simulink model "gm_uz_pmsm_model"  (R2023b)
settings: Solver=FixedStepAuto  StartTime=0.0  StopTime=0.05  RelTol=1e-3
PreLoadFcn:
  | uz_pmsm_model_init_parameter
PostLoadFcn:
  | % Import the data from Excel for a lookup table
  | FluxMapData = readtable('C:\Users\Philipp\ultrazohm\ultrazohm_sw\ip_cores\uz_pmsm_model\FluxMapData_2023-05-26_13-07-57.csv');
  | % Row indices for lookup table
  | d_current_in_d_axis = FluxMapData(8:27,1:end);
  | % Column indices for lookup table
  | q_current_in_d_axis = FluxMapData(29:48,1:end);
  | % Output values for lookup table
  | d_Flux_d_axis = FluxMapData(50:69,1:end);
undefined symbols (not defined in the file or in its folder): ad1, ad2, ad3, ad4, ad5, ad6, aq1, aq2, aq3, aq4, aq5, aq6, d_current_d_Flux, d_current_q_Flux, entkopplung_dynamic, entkopplung_linear, entkopplung_static, Fid1_Giq1, Fid2_Giq2, Flux_d, Flux_q, friction_coefficient, inertia, Ki_Bo_d, Ki_Bo_q, Kp_Bo_d, Kp_Bo_q, L_d, L_q, Ldq, parameter_nachfuerung, polepair, praediktion_entkopplung_nonlinear, psi_pm, q_current_d_Flux, q_current_q_Flux, R_1, simulate_mechanical, simulate_nonlinear_modell, simulate_open_loop, static_friction_torque, tau_sum, ts_regler
libraries: hdlmdlgenlib x21, slpidlib x6
(part 4 of 4)

== system gm_uz_pmsm_model/uz_pmsm_model/Sum23 ==
  In1 : Inport
  In2 : Inport  Port=2
  Sum23 : Sum  Inputs=+-  OutDataTypeStr=single  SampleTime=1e-08
  Sum23_pd1 : Delay  DelayLength=6
  Out1 : Outport
  wires:
  In1/1 -> Sum23/1
  In2/1 -> Sum23/2
  Sum23/1 -> Sum23_pd1/1
  Sum23_pd1/1 -> Out1/1

== system gm_uz_pmsm_model/uz_pmsm_model/Sum3 ==
  In1 : Inport
  In2 : Inport  Port=2
  Sum3 : Sum  Inputs=+-  OutDataTypeStr=single  SampleTime=1e-08
  Sum3_pd1 : Delay  DelayLength=6
  Out1 : Outport
  wires:
  In1/1 -> Sum3/1
  In2/1 -> Sum3/2
  Sum3/1 -> Sum3_pd1/1
  Sum3_pd1/1 -> Out1/1

== system gm_uz_pmsm_model/uz_pmsm_model/Sum31 ==
  In1 : Inport
  In2 : Inport  Port=2
  Sum31 : Sum  Inputs=+-  OutDataTypeStr=single  SampleTime=1e-08
  Sum31_pd1 : Delay  DelayLength=6
  Out1 : Outport
  wires:
  In1/1 -> Sum31/1
  In2/1 -> Sum31/2
  Sum31/1 -> Sum31_pd1/1
  Sum31_pd1/1 -> Out1/1

== system gm_uz_pmsm_model/uz_pmsm_model/Sum32 ==
  In1 : Inport
  In2 : Inport  Port=2
  Sum32 : Sum  OutDataTypeStr=single  SampleTime=1e-08
  Sum32_pd1 : Delay  DelayLength=6
  Out1 : Outport
  wires:
  In1/1 -> Sum32/1
  In2/1 -> Sum32/2
  Sum32/1 -> Sum32_pd1/1
  Sum32_pd1/1 -> Out1/1

== system gm_uz_pmsm_model/uz_pmsm_model/Sum33 ==
  In1 : Inport
  In2 : Inport  Port=2
  Sum33 : Sum  Inputs=+-  OutDataTypeStr=single  SampleTime=1e-08
  Sum33_pd1 : Delay  DelayLength=6
  Out1 : Outport
  wires:
  In1/1 -> Sum33/1
  In2/1 -> Sum33/2
  Sum33/1 -> Sum33_pd1/1
  Sum33_pd1/1 -> Out1/1

== system gm_uz_pmsm_model/uz_pmsm_model/Sum3_stage2 ==
  In1 : Inport
  In2 : Inport  Port=2
  Sum3_stage2 : Sum  OutDataTypeStr=single  SampleTime=1e-08
  Sum3_stage2_pd1 : Delay  DelayLength=6
  Out1 : Outport
  wires:
  In1/1 -> Sum3_stage2/1
  In2/1 -> Sum3_stage2/2
  Sum3_stage2/1 -> Sum3_stage2_pd1/1
  Sum3_stage2_pd1/1 -> Out1/1

== system gm_uz_pmsm_model/uz_pmsm_model/Sum3_stage21 ==
  In1 : Inport
  In2 : Inport  Port=2
  Sum3_stage21 : Sum  Inputs=+-  OutDataTypeStr=single  SampleTime=1e-08
  Sum3_stage21_pd1 : Delay  DelayLength=6
  Out1 : Outport
  wires:
  In1/1 -> Sum3_stage21/1
  In2/1 -> Sum3_stage21/2
  Sum3_stage21/1 -> Sum3_stage21_pd1/1
  Sum3_stage21_pd1/1 -> Out1/1

== system gm_uz_pmsm_model/uz_pmsm_model/Sum3_stage3 ==
  In1 : Inport
  In2 : Inport  Port=2
  Sum3_stage3 : Sum  Inputs=+-  OutDataTypeStr=single  SampleTime=1e-08
  Sum3_stage3_pd1 : Delay  DelayLength=6
  Out1 : Outport
  wires:
  In1/1 -> Sum3_stage3/1
  In2/1 -> Sum3_stage3/2
  Sum3_stage3/1 -> Sum3_stage3_pd1/1
  Sum3_stage3_pd1/1 -> Out1/1

== system gm_uz_pmsm_model/uz_pmsm_model/Sum3_stage31 ==
  In1 : Inport
  In2 : Inport  Port=2
  Sum3_stage31 : Sum  Inputs=+-  OutDataTypeStr=single  SampleTime=1e-08
  Sum3_stage31_pd1 : Delay  DelayLength=6
  Out1 : Outport
  wires:
  In1/1 -> Sum3_stage31/1
  In2/1 -> Sum3_stage31/2
  Sum3_stage31/1 -> Sum3_stage31_pd1/1
  Sum3_stage31_pd1/1 -> Out1/1

== system gm_uz_pmsm_model/uz_pmsm_model/Sum3_stage4 ==
  In1 : Inport
  In2 : Inport  Port=2
  Sum3_stage4 : Sum  OutDataTypeStr=single  SampleTime=1e-08
  Sum3_stage4_pd1 : Delay  DelayLength=6
  Out1 : Outport
  wires:
  In1/1 -> Sum3_stage4/1
  In2/1 -> Sum3_stage4/2
  Sum3_stage4/1 -> Sum3_stage4_pd1/1
  Sum3_stage4_pd1/1 -> Out1/1

== system gm_uz_pmsm_model/uz_pmsm_model/Sum4 ==
  In1 : Inport
  In2 : Inport  Port=2
  Sum4 : Sum  Inputs=+-  OutDataTypeStr=single  SampleTime=1e-08
  Sum4_pd1 : Delay  DelayLength=6
  Out1 : Outport
  wires:
  In1/1 -> Sum4/1
  In2/1 -> Sum4/2
  Sum4/1 -> Sum4_pd1/1
  Sum4_pd1/1 -> Out1/1

== system gm_uz_pmsm_model/uz_pmsm_model/Sum41 ==
  In1 : Inport
  In2 : Inport  Port=2
  Sum41 : Sum  OutDataTypeStr=single  SampleTime=1e-08
  Sum41_pd1 : Delay  DelayLength=6
  Out1 : Outport
  wires:
  In1/1 -> Sum41/1
  In2/1 -> Sum41/2
  Sum41/1 -> Sum41_pd1/1
  Sum41_pd1/1 -> Out1/1

== system gm_uz_pmsm_model/uz_pmsm_model/Sum42 ==
  In1 : Inport
  In2 : Inport  Port=2
  Sum42 : Sum  OutDataTypeStr=single  SampleTime=1e-08
  Sum42_pd1 : Delay  DelayLength=6
  Out1 : Outport
  wires:
  In1/1 -> Sum42/1
  In2/1 -> Sum42/2
  Sum42/1 -> Sum42_pd1/1
  Sum42_pd1/1 -> Out1/1

== system gm_uz_pmsm_model/uz_pmsm_model/Sum4_stage2 ==
  In1 : Inport
  In2 : Inport  Port=2
  Sum4_stage2 : Sum  Inputs=+-  OutDataTypeStr=single  SampleTime=1e-08
  Sum4_stage2_pd1 : Delay  DelayLength=6
  Out1 : Outport
  wires:
  In1/1 -> Sum4_stage2/1
  In2/1 -> Sum4_stage2/2
  Sum4_stage2/1 -> Sum4_stage2_pd1/1
  Sum4_stage2_pd1/1 -> Out1/1

== system gm_uz_pmsm_model/uz_pmsm_model/Sum4_stage3 ==
  In1 : Inport
  In2 : Inport  Port=2
  Sum4_stage3 : Sum  Inputs=+-  OutDataTypeStr=single  SampleTime=1e-08
  Sum4_stage3_pd1 : Delay  DelayLength=6
  Out1 : Outport
  wires:
  In1/1 -> Sum4_stage3/1
  In2/1 -> Sum4_stage3/2
  Sum4_stage3/1 -> Sum4_stage3_pd1/1
  Sum4_stage3_pd1/1 -> Out1/1

== system gm_uz_pmsm_model/uz_pmsm_model/Sum4_stage4 ==
  In1 : Inport
  In2 : Inport  Port=2
  Sum4_stage4 : Sum  Inputs=+-  OutDataTypeStr=single  SampleTime=1e-08
  Sum4_stage4_pd1 : Delay  DelayLength=6
  Out1 : Outport
  wires:
  In1/1 -> Sum4_stage4/1
  In2/1 -> Sum4_stage4/2
  Sum4_stage4/1 -> Sum4_stage4_pd1/1
  Sum4_stage4_pd1/1 -> Out1/1

== system gm_uz_pmsm_model/uz_pmsm_model/Sum5 ==
  In1 : Inport
  In2 : Inport  Port=2
  Sum5 : Sum  Inputs=+-  OutDataTypeStr=single  SampleTime=1e-08
  Sum5_pd1 : Delay  DelayLength=6
  Out1 : Outport
  wires:
  In1/1 -> Sum5/1
  In2/1 -> Sum5/2
  Sum5/1 -> Sum5_pd1/1
  Sum5_pd1/1 -> Out1/1

== system gm_uz_pmsm_model/uz_pmsm_model/Sum51 ==
  In1 : Inport
  In2 : Inport  Port=2
  Sum51 : Sum  OutDataTypeStr=single  SampleTime=1e-08
  Sum51_pd1 : Delay  DelayLength=6
  Out1 : Outport
  wires:
  In1/1 -> Sum51/1
  In2/1 -> Sum51/2
  Sum51/1 -> Sum51_pd1/1
  Sum51_pd1/1 -> Out1/1

== system gm_uz_pmsm_model/uz_pmsm_model/Sum52 ==
  In1 : Inport
  In2 : Inport  Port=2
  Sum52 : Sum  OutDataTypeStr=single  SampleTime=1e-08
  Sum52_pd1 : Delay  DelayLength=6
  Out1 : Outport
  wires:
  In1/1 -> Sum52/1
  In2/1 -> Sum52/2
  Sum52/1 -> Sum52_pd1/1
  Sum52_pd1/1 -> Out1/1

== system gm_uz_pmsm_model/uz_pmsm_model/Sum53 ==
  In1 : Inport
  In2 : Inport  Port=2
  Sum53 : Sum  OutDataTypeStr=single  SampleTime=1e-08
  Sum53_pd1 : Delay  DelayLength=6
  Out1 : Outport
  wires:
  In1/1 -> Sum53/1
  In2/1 -> Sum53/2
  Sum53/1 -> Sum53_pd1/1
  Sum53_pd1/1 -> Out1/1

== system gm_uz_pmsm_model/uz_pmsm_model/Sum6 ==
  In1 : Inport
  In2 : Inport  Port=2
  Sum6 : Sum  Inputs=+-  OutDataTypeStr=single  SampleTime=1e-08
  Sum6_pd1 : Delay  DelayLength=6
  Out1 : Outport
  wires:
  In1/1 -> Sum6/1
  In2/1 -> Sum6/2
  Sum6/1 -> Sum6_pd1/1
  Sum6_pd1/1 -> Out1/1

== system gm_uz_pmsm_model/uz_pmsm_model/Sum7 ==
  In1 : Inport
  In2 : Inport  Port=2
  Sum7 : Sum  Inputs=+-  OutDataTypeStr=single  SampleTime=1e-08
  Sum7_pd1 : Delay  DelayLength=6
  Out1 : Outport
  wires:
  In1/1 -> Sum7/1
  In2/1 -> Sum7/2
  Sum7/1 -> Sum7_pd1/1
  Sum7_pd1/1 -> Out1/1

== system gm_uz_pmsm_model/uz_pmsm_model/Sum71 ==
  In1 : Inport
  In2 : Inport  Port=2
  Sum71 : Sum  Inputs=+-  OutDataTypeStr=single  SampleTime=1e-08
  Sum71_pd1 : Delay  DelayLength=6
  Out1 : Outport
  wires:
  In1/1 -> Sum71/1
  In2/1 -> Sum71/2
  Sum71/1 -> Sum71_pd1/1
  Sum71_pd1/1 -> Out1/1

== system gm_uz_pmsm_model/uz_pmsm_model/Sum8 ==
  In1 : Inport
  In2 : Inport  Port=2
  Sum8 : Sum  Inputs=+-  OutDataTypeStr=single  SampleTime=1e-08
  Sum8_pd1 : Delay  DelayLength=6
  Out1 : Outport
  wires:
  In1/1 -> Sum8/1
  In2/1 -> Sum8/2
  Sum8/1 -> Sum8_pd1/1
  Sum8_pd1/1 -> Out1/1

== system gm_uz_pmsm_model/uz_pmsm_model/Tanh ==
  In1 : Inport
  Tanh : Trigonometry  Operator=tanh  SampleTime=1e-08
  Tanh_pd1 : Delay  DelayLength=25
  Out1 : Outport
  wires:
  In1/1 -> Tanh/1
  Tanh/1 -> Tanh_pd1/1
  Tanh_pd1/1 -> Out1/1

== system gm_uz_pmsm_model/uz_pmsm_model/Tanh1 ==
  In1 : Inport
  Tanh1 : Trigonometry  Operator=cosh  SampleTime=1e-08
  Tanh1_pd1 : Delay  DelayLength=17
  Out1 : Outport
  wires:
  In1/1 -> Tanh1/1
  Tanh1/1 -> Tanh1_pd1/1
  Tanh1_pd1/1 -> Out1/1

== system gm_uz_pmsm_model/uz_pmsm_model/Tanh11 ==
  In1 : Inport
  Tanh11 : Trigonometry  Operator=tanh  SampleTime=1e-08
  Tanh11_pd1 : Delay  DelayLength=25
  Out1 : Outport
  wires:
  In1/1 -> Tanh11/1
  Tanh11/1 -> Tanh11_pd1/1
  Tanh11_pd1/1 -> Out1/1

== system gm_uz_pmsm_model/uz_pmsm_model/Tanh12 ==
  In1 : Inport
  Tanh12 : Trigonometry  Operator=tanh  SampleTime=1e-08
  Tanh12_pd1 : Delay  DelayLength=25
  Out1 : Outport
  wires:
  In1/1 -> Tanh12/1
  Tanh12/1 -> Tanh12_pd1/1
  Tanh12_pd1/1 -> Out1/1

== system gm_uz_pmsm_model/uz_pmsm_model/Tanh13 ==
  In1 : Inport
  Tanh13 : Trigonometry  Operator=cosh  SampleTime=1e-08
  Tanh13_pd1 : Delay  DelayLength=17
  Out1 : Outport
  wires:
  In1/1 -> Tanh13/1
  Tanh13/1 -> Tanh13_pd1/1
  Tanh13_pd1/1 -> Out1/1

== system gm_uz_pmsm_model/uz_pmsm_model/Tanh2 ==
  In1 : Inport
  Tanh2 : Trigonometry  Operator=cosh  SampleTime=1e-08
  Tanh2_pd1 : Delay  DelayLength=17
  Out1 : Outport
  wires:
  In1/1 -> Tanh2/1
  Tanh2/1 -> Tanh2_pd1/1
  Tanh2_pd1/1 -> Out1/1

== system gm_uz_pmsm_model/uz_pmsm_model/Tanh21 ==
  In1 : Inport
  Tanh21 : Trigonometry  Operator=cosh  SampleTime=1e-08
  Tanh21_pd1 : Delay  DelayLength=17
  Out1 : Outport
  wires:
  In1/1 -> Tanh21/1
  Tanh21/1 -> Tanh21_pd1/1
  Tanh21_pd1/1 -> Out1/1

== system gm_uz_pmsm_model/uz_pmsm_model/Tanh3 ==
  In1 : Inport
  Tanh3 : Trigonometry  Operator=cosh  SampleTime=1e-08
  Tanh3_pd1 : Delay  DelayLength=17
  Out1 : Outport
  wires:
  In1/1 -> Tanh3/1
  Tanh3/1 -> Tanh3_pd1/1
  Tanh3_pd1/1 -> Out1/1

== system gm_uz_pmsm_model/uz_pmsm_model/Tanh31 ==
  In1 : Inport
  Tanh31 : Trigonometry  Operator=cosh  SampleTime=1e-08
  Tanh31_pd1 : Delay  DelayLength=17
  Out1 : Outport
  wires:
  In1/1 -> Tanh31/1
  Tanh31/1 -> Tanh31_pd1/1
  Tanh31_pd1/1 -> Out1/1

== system gm_uz_pmsm_model/uz_pmsm_model/Tanh4 ==
  In1 : Inport
  Tanh4 : Trigonometry  Operator=cosh  SampleTime=1e-08
  Tanh4_pd1 : Delay  DelayLength=17
  Out1 : Outport
  wires:
  In1/1 -> Tanh4/1
  Tanh4/1 -> Tanh4_pd1/1
  Tanh4_pd1/1 -> Out1/1

== system gm_uz_pmsm_model/uz_pmsm_model/Tanh41 ==
  In1 : Inport
  Tanh41 : Trigonometry  Operator=cosh  SampleTime=1e-08
  Tanh41_pd1 : Delay  DelayLength=17
  Out1 : Outport
  wires:
  In1/1 -> Tanh41/1
  Tanh41/1 -> Tanh41_pd1/1
  Tanh41_pd1/1 -> Out1/1

== system gm_uz_pmsm_model/uz_pmsm_model/Tanh5 ==
  In1 : Inport
  Tanh5 : Trigonometry  Operator=tanh  SampleTime=1e-08
  Tanh5_pd1 : Delay  DelayLength=25
  Out1 : Outport
  wires:
  In1/1 -> Tanh5/1
  Tanh5/1 -> Tanh5_pd1/1
  Tanh5_pd1/1 -> Out1/1

== system gm_uz_pmsm_model/Curren t_Controller_With_FluxMaps_OLD/Entkopplungen/Lineare_Entkopplung ==
  i_d : Inport
  i_q : Inport  Port=2
  omega_m : Inport  Port=3
  Constant1 : Constant  Value=psi_pm  SampleTime=-1
  Gain : Gain  Gain=L_q
  Gain1 : Gain  Gain=L_d
  Gain2 : Gain  Gain=polepair
  Product : Product
  Product1 : Product
  Sum6 : Sum  Inputs=|++
  u_d : Outport
  u_q : Outport  Port=2
  wires:
  Gain/1 -> Product/1
  Gain2/1 -> Product/2, Product1/2
  Gain1/1 -> Sum6/1
  Product1/1 -> u_q/1
  i_q/1 -> Gain/1
  Constant1/1 -> Sum6/2
  i_d/1 -> Gain1/1
  Product/1 -> u_d/1
  Sum6/1 -> Product1/1
  omega_m/1 -> Gain2/1

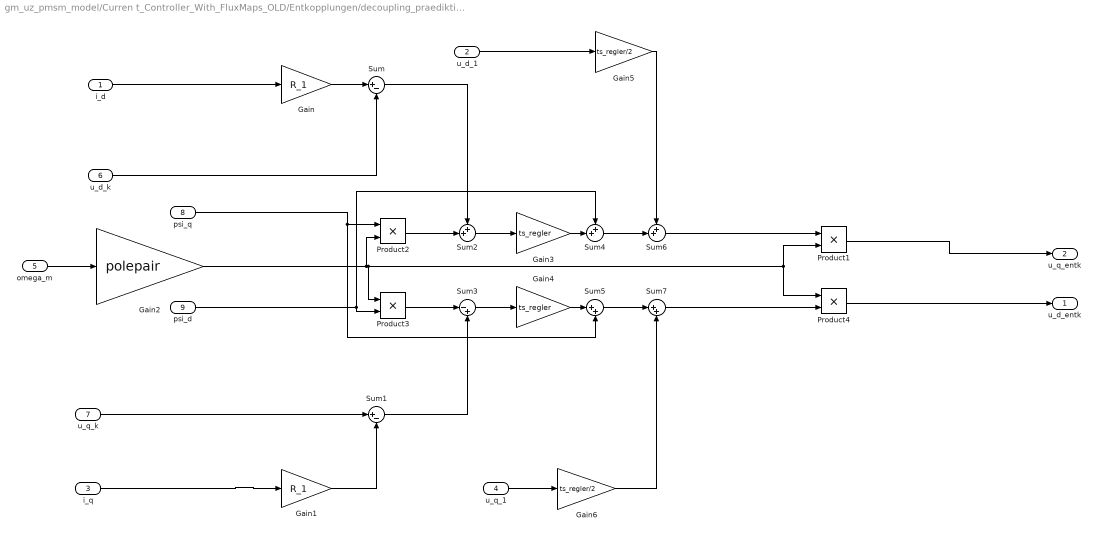
== system gm_uz_pmsm_model/Curren t_Controller_With_FluxMaps_OLD/Entkopplungen/decoupling_praediktion ==
  i_d : Inport
  u_d_1 : Inport  Port=2
  i_q : Inport  Port=3
  u_q_1 : Inport  Port=4
  omega_m : Inport  Port=5
  u_d_k : Inport  Port=6
  u_q_k : Inport  Port=7
  psi_q : Inport  Port=8
  psi_d : Inport  Port=9
  Gain : Gain  Gain=R_1
  Gain1 : Gain  Gain=R_1
  Gain2 : Gain  Gain=polepair
  Gain3 : Gain  Gain=ts_regler
  Gain4 : Gain  Gain=ts_regler
  Gain5 : Gain  Gain=ts_regler/2
  Gain6 : Gain  Gain=ts_regler/2
  Product{1..4} (4 alike) : Product
  Sum : Sum  Inputs=|+-
  Sum1 : Sum  Inputs=|+-
  Sum2 : Sum  Inputs=++|
  Sum3 : Sum  Inputs=|-+
  Sum4 : Sum  Inputs=++|
  Sum5 : Sum  Inputs=|++
  Sum6 : Sum  Inputs=++|
  Sum7 : Sum  Inputs=|++
  u_d_entk : Outport
  u_q_entk : Outport  Port=2
  wires:
  Product4/1 -> u_d_entk/1
  Product1/1 -> u_q_entk/1
  i_q/1 -> Gain1/1
  i_d/1 -> Gain/1
  omega_m/1 -> Gain2/1
  Sum7/1 -> Product4/2
  Sum6/1 -> Product1/1
  Gain6/1 -> Sum7/2
  Sum5/1 -> Sum7/1
  Gain5/1 -> Sum6/1
  u_q_1/1 -> Gain6/1
  Sum4/1 -> Sum6/2
  u_d_1/1 -> Gain5/1
  Gain4/1 -> Sum5/1
  Gain3/1 -> Sum4/2
  Sum2/1 -> Gain3/1
  Sum3/1 -> Gain4/1
  Sum1/1 -> Sum3/2
  Sum/1 -> Sum2/1
  Product2/1 -> Sum2/2
  Product3/1 -> Sum3/1
  Gain1/1 -> Sum1/2
  u_q_k/1 -> Sum1/1
  Gain/1 -> Sum/1
  u_d_k/1 -> Sum/2
  Gain2/1 -> Product2/2, Product3/1, Product4/1, Product1/2
  psi_d/1 -> Sum4/1, Product3/2
  psi_q/1 -> Product2/1, Sum5/2

== system gm_uz_pmsm_model/Curren t_Controller_With_FluxMaps_OLD/Entkopplungen/dynamic_nonlinear_entkopplung1 ==
  i_d : Inport
  i_q : Inport  Port=2
  psi_d : Inport  Port=3
  psi_q : Inport  Port=4
  Ldq_LUT : Inport  Port=5
  Lqd_LUT : Inport  Port=6
  omega_m : Inport  Port=7
  Gain2 : Gain  Gain=polepair
  Product{,1..3} (4 alike) : Product
  Sum1 : Sum  Inputs=++|
  Sum6 : Sum  Inputs=++|
  u_d : Outport
  u_q : Outport  Port=2
  wires:
  Product2/1 -> Sum1/1
  Product3/1 -> Sum6/1
  Lqd_LUT/1 -> Product3/2
  i_q/1 -> Product3/1
  Sum1/1 -> u_d/1
  Product/1 -> Sum1/2
  Product1/1 -> Sum6/2
  Sum6/1 -> u_q/1
  Ldq_LUT/1 -> Product2/2
  i_d/1 -> Product2/1
  omega_m/1 -> Gain2/1
  psi_d/1 -> Product1/1  "psi_d_LUT"
  Gain2/1 -> Product/2, Product1/2
  psi_q/1 -> Product/1  "psi_q_LUT"

== system gm_uz_pmsm_model/Curren t_Controller_With_FluxMaps_OLD/Entkopplungen/static_nonlinear_entkopplung ==
  psi_d : Inport
  psi_q : Inport  Port=2
  omega_m : Inport  Port=3
  Gain2 : Gain  Gain=polepair
  Product : Product  OutDataTypeStr=Inherit: Same as first input
  Product1 : Product
  Scope : Scope  NumInputPorts=2
  u_d : Outport
  u_q : Outport  Port=2
  wires:
  omega_m/1 -> Gain2/1
  psi_d/1 -> Product1/1  "psi_d_LUT"
  Product/1 -> u_d/1, Scope/2
  Product1/1 -> u_q/1, Scope/1
  Gain2/1 -> Product/2, Product1/2
  psi_q/1 -> Product/1  "psi_q_LUT"

== system gm_uz_pmsm_model/Curren t_Controller_With_FluxMaps_OLD/Psi_d_q/Ldd_approx1 ==
  psiq_cross_s1_integrated : Inport
  Id : Inport  Port=2
  FittingParameters : Inport  Port=3
  Demux : Demux  Outputs=23
  Product{,1..3} (4 alike) : Product  OutDataTypeStr=single
  Product10 : Product  Inputs=3  OutDataTypeStr=single
  Product14 : Product
  Product15 : Product
  Reciprocal : Product  Inputs=/  RndMeth=Zero  SaturateOnIntegerOverflow=on
  Reciprocal1 : Product  Inputs=/  RndMeth=Zero  SaturateOnIntegerOverflow=on
  Sum : Sum  Inputs=|+-  OutDataTypeStr=single
  Sum1 : Sum  Inputs=|+-  OutDataTypeStr=single
  Sum2 : Sum  Inputs=|+-
  Sum7 : Sum  Inputs=|+-
  Tanh1 : Trigonometry  Operator=cosh
  Tanh4 : Trigonometry  Operator=cosh
  Ldd : Outport
  wires:
  Demux/16 -> Product1/2  "ad1*ad2"
  Demux/15 -> Product3/2  "ad4*ad5"
  Reciprocal/1 -> Product1/1
  psiq_cross_s1_integrated/1 -> Product10/2
  Product2/1 -> Tanh1/1
  Product/1 -> Tanh4/1
  Product14/1 -> Reciprocal/1
  Product15/1 -> Reciprocal1/1
  Reciprocal1/1 -> Product3/1
  Tanh1/1 -> Product15/1, Product15/2
  Tanh4/1 -> Product14/2, Product14/1
  Demux/13 -> Product10/3  "F1G1"
  Sum7/1 -> Ldd/1  "psid_cross_s1"
  Product10/1 -> Sum7/2  "psid_cross"
  Sum2/1 -> Product10/1  "psid_cross_s1_abgeleitet"
  Product3/1 -> Sum2/2  "psid_s1"
  Id/1 -> Sum/1, Sum1/1
  Demux/6 -> Sum1/2  "ad6"
  Demux/5 -> Product2/2  "ad5"
  Sum1/1 -> Product2/1
  Product1/1 -> Sum2/1, Sum7/1  "psidself_abgeleitet"
  Demux/2 -> Product/2  "ad2"
  Sum/1 -> Product/1
  Demux/3 -> Sum/2  "ad3"
  FittingParameters/1 -> Demux/1

== system gm_uz_pmsm_model/Curren t_Controller_With_FluxMaps_OLD/Psi_d_q/Lqq_approx1 ==
  psid_cross_s1_integrated : Inport
  Iq : Inport  Port=2
  FittingParameters : Inport  Port=3
  Demux : Demux  Outputs=23
  Product : Product  OutDataTypeStr=Inherit: Same as first input
  Product1 : Product
  Product14 : Product  OutDataTypeStr=Inherit: Same as first input
  Product15 : Product
  Product2 : Product  OutDataTypeStr=Inherit: Same as first input
  Product20 : Product  Inputs=3
  Product3 : Product
  Reciprocal : Product  Inputs=/  RndMeth=Zero  SaturateOnIntegerOverflow=on
  Reciprocal1 : Product  Inputs=/  RndMeth=Zero  SaturateOnIntegerOverflow=on
  Sum1 : Sum  Inputs=|++
  Sum10 : Sum  Inputs=|+-
  Sum2 : Sum  Inputs=|+-
  Sum4 : Sum  Inputs=|++
  Tanh1 : Trigonometry  Operator=cosh
  Tanh3 : Trigonometry  Operator=cosh
  Lqq : Outport
  wires:
  Demux/17 -> Product3/2  "aq4*aq5"
  Demux/18 -> Product1/2  "aq1*aq2"
  psid_cross_s1_integrated/1 -> Product20/2
  Product14/1 -> Reciprocal/1
  Product/1 -> Tanh3/1
  Product2/1 -> Tanh1/1
  Product15/1 -> Reciprocal1/1
  Product3/1 -> Sum4/1  "psid_s1"
  Sum4/1 -> Sum2/2
  Sum1/1 -> Sum2/1, Sum10/1
  Product1/1 -> Sum1/1  "psidself_abgeleitet"
  Demux/11 -> Product2/2  "aq5"
  Iq/1 -> Product/1, Product2/1
  Demux/8 -> Product/2  "aq2"
  Reciprocal1/1 -> Product3/1
  Reciprocal/1 -> Product1/1
  Sum2/1 -> Product20/1
  Tanh1/1 -> Product15/1, Product15/2
  Tanh3/1 -> Product14/2, Product14/1
  Demux/9 -> Sum1/2  "aq3"
  Demux/14 -> Product20/3
  Sum10/1 -> Lqq/1  "Lqq"
  Product20/1 -> Sum10/2  "psiq_cross"
  Demux/12 -> Sum4/2  "aq6"
  FittingParameters/1 -> Demux/1

== system gm_uz_pmsm_model/Curren t_Controller_With_FluxMaps_OLD/Psi_d_q/psid_approx ==
  Id : Inport
  Iq : Inport  Port=2
  FittingParameters : Inport  Port=3
  Demux : Demux  Outputs=23
  Log : Math  Operator=log  SignedPower=on
  Log1 : Math  Operator=log  SignedPower=on
  Product{,1..2,4..5,8} (6 alike) : Product  OutDataTypeStr=Inherit: Same as first input
  Product10 : Product  Inputs=3
  Product{3,6..7,12} (4 alike) : Product
  Sum : Sum  Inputs=|+-  OutDataTypeStr=Inherit: Same as first input
  Sum1 : Sum  Inputs=|+-
  Sum2 : Sum  Inputs=|+-  OutDataTypeStr=Inherit: Same as first input
  Sum3 : Sum  Inputs=|++-  OutDataTypeStr=Inherit: Same as first input
  Sum7 : Sum  Inputs=|+-  OutDataTypeStr=Inherit: Same as first input
  Tanh : Trigonometry  Operator=tanh
  Tanh1 : Trigonometry  Operator=tanh
  Tanh2 : Trigonometry  Operator=cosh
  Tanh3 : Trigonometry  Operator=cosh
  Terminator : Terminator
  psid : Outport
  psiq_cross_s1_integrated : Outport  Port=2
  wires:
  Demux/23 -> Product7/2
  Product5/1 -> Tanh3/1
  Product4/1 -> Tanh2/1
  Product2/1 -> Tanh1/1
  Product/1 -> Tanh/1
  Tanh1/1 -> Product3/1
  Tanh/1 -> Product1/1
  Log1/1 -> Product12/1
  Log/1 -> Product6/1
  Demux/13 -> Product10/3  "Reciprodical_F1G1"
  Demux/14 -> Terminator/1
  Sum7/1 -> psid/1  "psi_d_approx"
  Product10/1 -> Sum7/2  "psid_cross"
  Demux/8 -> Product4/2  "aq2"
  Demux/11 -> Product5/2  "aq5"
  Sum3/1 -> psiq_cross_s1_integrated/1, Product10/2  "psiq_cross_s1_integrated"
  Product12/1 -> Sum3/3
  Demux/19 -> Product12/2
  Product6/1 -> Sum3/1
  Demux/20 -> Product6/2
  Product7/1 -> Sum3/2
  Product8/1 -> Product7/1
  Tanh3/1 -> Log1/1
  Tanh2/1 -> Log/1
  Sum2/1 -> Product10/1  "psid_cross_s1"
  Iq/1 -> Product4/1, Product5/1, Product8/1, Product8/2
  Product3/1 -> Sum2/2  "psid_s1"
  Id/1 -> Sum/1, Sum1/1
  Demux/6 -> Sum1/2  "ad6"
  Demux/5 -> Product2/2  "ad5"
  Sum1/1 -> Product2/1
  Demux/4 -> Product3/2  "ad4"
  Product1/1 -> Sum2/1, Sum7/1  "psidself"
  Demux/2 -> Product/2  "ad2"
  Sum/1 -> Product/1
  Demux/3 -> Sum/2  "ad3"
  Demux/1 -> Product1/2  "ad1"
  FittingParameters/1 -> Demux/1

== system gm_uz_pmsm_model/Curren t_Controller_With_FluxMaps_OLD/Psi_d_q/psid_approx1 ==
  Id : Inport
  Iq : Inport  Port=2
  FittingParameters : Inport  Port=3
  Demux : Demux  Outputs=23
  Log : Math  Operator=log  SignedPower=on
  Log1 : Math  Operator=log  SignedPower=on
  Product{,1..2,4..5,8} (6 alike) : Product  OutDataTypeStr=Inherit: Same as first input
  Product10 : Product  Inputs=3
  Product{3,6..7,12} (4 alike) : Product
  Sum : Sum  Inputs=|+-  OutDataTypeStr=Inherit: Same as first input
  Sum1 : Sum  Inputs=|+-
  Sum2 : Sum  Inputs=|+-  OutDataTypeStr=Inherit: Same as first input
  Sum3 : Sum  Inputs=|++-  OutDataTypeStr=Inherit: Same as first input
  Sum7 : Sum  Inputs=|+-  OutDataTypeStr=Inherit: Same as first input
  Tanh : Trigonometry  Operator=tanh
  Tanh1 : Trigonometry  Operator=tanh
  Tanh2 : Trigonometry  Operator=cosh
  Tanh3 : Trigonometry  Operator=cosh
  Terminator : Terminator
  psid : Outport
  psiq_cross_s1_integrated : Outport  Port=2
  wires:
  Demux/23 -> Product7/2
  Product5/1 -> Tanh3/1
  Product4/1 -> Tanh2/1
  Product2/1 -> Tanh1/1
  Product/1 -> Tanh/1
  Tanh1/1 -> Product3/1
  Tanh/1 -> Product1/1
  Log1/1 -> Product12/1
  Log/1 -> Product6/1
  Demux/13 -> Product10/3  "Reciprodical_F1G1"
  Demux/14 -> Terminator/1
  Sum7/1 -> psid/1  "psi_d_approx"
  Product10/1 -> Sum7/2  "psid_cross"
  Demux/8 -> Product4/2  "aq2"
  Demux/11 -> Product5/2  "aq5"
  Sum3/1 -> psiq_cross_s1_integrated/1, Product10/2  "psiq_cross_s1_integrated"
  Product12/1 -> Sum3/3
  Demux/19 -> Product12/2
  Product6/1 -> Sum3/1
  Demux/20 -> Product6/2
  Product7/1 -> Sum3/2
  Product8/1 -> Product7/1
  Tanh3/1 -> Log1/1
  Tanh2/1 -> Log/1
  Sum2/1 -> Product10/1  "psid_cross_s1"
  Iq/1 -> Product4/1, Product5/1, Product8/1, Product8/2
  Product3/1 -> Sum2/2  "psid_s1"
  Id/1 -> Sum/1, Sum1/1
  Demux/6 -> Sum1/2  "ad6"
  Demux/5 -> Product2/2  "ad5"
  Sum1/1 -> Product2/1
  Demux/4 -> Product3/2  "ad4"
  Product1/1 -> Sum2/1, Sum7/1  "psidself"
  Demux/2 -> Product/2  "ad2"
  Sum/1 -> Product/1
  Demux/3 -> Sum/2  "ad3"
  Demux/1 -> Product1/2  "ad1"
  FittingParameters/1 -> Demux/1

== system gm_uz_pmsm_model/Curren t_Controller_With_FluxMaps_OLD/Psi_d_q/psiq_approx ==
  Id : Inport
  Iq : Inport  Port=2
  FittingParameters : Inport  Port=3
  Demux : Demux  Outputs=23
  Log1 : Math  Operator=log  SignedPower=on
  Log2 : Math  Operator=log  SignedPower=on
  Product{,2,7,10} (4 alike) : Product  OutDataTypeStr=Inherit: Same as first input
  Product{1,3..6,9} (6 alike) : Product
  Product20 : Product  Inputs=3
  Sum1 : Sum  Inputs=|++
  Sum10 : Sum  Inputs=|+-
  Sum2 : Sum  Inputs=|+-
  Sum3 : Sum  Inputs=-+|
  Sum4 : Sum  Inputs=++|
  Sum5 : Sum  Inputs=|+-
  Sum6 : Sum  Inputs=-+|
  Tanh : Trigonometry  Operator=tanh
  Tanh1 : Trigonometry  Operator=tanh
  Tanh2 : Trigonometry  Operator=cosh
  Tanh4 : Trigonometry  Operator=cosh
  psiq : Outport
  psid_cross_s1_integrated : Outport  Port=2
  wires:
  Product/1 -> Tanh/1
  Product2/1 -> Tanh1/1
  Tanh/1 -> Product1/1
  Tanh1/1 -> Product3/1
  Log2/1 -> Product4/2
  Log1/1 -> Product9/2
  Demux/14 -> Product20/3
  Sum10/1 -> psiq/1  "psiq_approx"
  Product20/1 -> Sum10/2  "psiq_cross"
  Sum5/1 -> Product20/2, psid_cross_s1_integrated/1  "psid_cross_s1_integrated"
  Id/1 -> Sum3/2, Sum6/2
  Demux/6 -> Sum6/1  "ad6"
  Demux/5 -> Product10/1  "ad5"
  Demux/2 -> Product7/1  "ad2"
  Demux/3 -> Sum3/1  "ad3"
  Sum6/1 -> Product10/2  "psid_cross_s1"
  Demux/21 -> Product9/1
  Tanh2/1 -> Log1/1
  Product10/1 -> Tanh2/1  "psid_s1"
  Product9/1 -> Sum5/2
  Product4/1 -> Sum5/1
  Product7/1 -> Tanh4/1  "psid_s1"
  Sum3/1 -> Product7/2  "psid_cross_s1"
  Product6/1 -> Sum1/2
  Product3/1 -> Sum1/1  "psiq_s1"
  Sum1/1 -> Sum2/2
  Sum4/1 -> Sum2/1, Sum10/1  "psiq_self"
  Product5/1 -> Sum4/1
  Product1/1 -> Sum4/2
  Demux/22 -> Product4/1
  Tanh4/1 -> Log2/1
  Demux/9 -> Product5/2  "aq3"
  Iq/1 -> Product5/1, Product/1, Product6/1, Product2/1
  Demux/7 -> Product1/2  "aq1"
  Demux/11 -> Product2/2  "aq5"
  Demux/8 -> Product/2  "aq2"
  Demux/12 -> Product6/2  "aq6"
  Demux/10 -> Product3/2  "aq4"
  Sum2/1 -> Product20/1  "psiq_cross_s1"
  FittingParameters/1 -> Demux/1

== system gm_uz_pmsm_model/Curren t_Controller_With_FluxMaps_OLD/Psi_d_q/psiq_approx1 ==
  Id : Inport
  Iq : Inport  Port=2
  FittingParameters : Inport  Port=3
  Demux : Demux  Outputs=23
  Log1 : Math  Operator=log  SignedPower=on
  Log2 : Math  Operator=log  SignedPower=on
  Product{,2,7,10} (4 alike) : Product  OutDataTypeStr=Inherit: Same as first input
  Product{1,3..6,9} (6 alike) : Product
  Product20 : Product  Inputs=3
  Sum1 : Sum  Inputs=|++
  Sum10 : Sum  Inputs=|+-  OutDataTypeStr=Inherit: Same as first input
  Sum2 : Sum  Inputs=|+-
  Sum3 : Sum  Inputs=-+|
  Sum4 : Sum  Inputs=++|
  Sum5 : Sum  Inputs=|+-
  Sum6 : Sum  Inputs=-+|
  Tanh : Trigonometry  Operator=tanh
  Tanh1 : Trigonometry  Operator=tanh
  Tanh2 : Trigonometry  Operator=cosh
  Tanh4 : Trigonometry  Operator=cosh
  psiq : Outport
  psid_cross_s1_integrated : Outport  Port=2
  wires:
  Product/1 -> Tanh/1
  Product2/1 -> Tanh1/1
  Tanh/1 -> Product1/1
  Tanh1/1 -> Product3/1
  Log2/1 -> Product4/2
  Log1/1 -> Product9/2
  Demux/14 -> Product20/3
  Sum10/1 -> psiq/1  "psiq_approx"
  Product20/1 -> Sum10/2  "psiq_cross"
  Sum5/1 -> Product20/2, psid_cross_s1_integrated/1  "psid_cross_s1_integrated"
  Id/1 -> Sum3/2, Sum6/2
  Demux/6 -> Sum6/1  "ad6"
  Demux/5 -> Product10/1  "ad5"
  Demux/2 -> Product7/1  "ad2"
  Demux/3 -> Sum3/1  "ad3"
  Sum6/1 -> Product10/2  "psid_cross_s1"
  Demux/21 -> Product9/1
  Tanh2/1 -> Log1/1
  Product10/1 -> Tanh2/1  "psid_s1"
  Product9/1 -> Sum5/2
  Product4/1 -> Sum5/1
  Product7/1 -> Tanh4/1  "psid_s1"
  Sum3/1 -> Product7/2  "psid_cross_s1"
  Product6/1 -> Sum1/2
  Product3/1 -> Sum1/1  "psiq_s1"
  Sum1/1 -> Sum2/2
  Sum4/1 -> Sum2/1, Sum10/1  "psiq_self"
  Product5/1 -> Sum4/1
  Product1/1 -> Sum4/2
  Demux/22 -> Product4/1
  Tanh4/1 -> Log2/1
  Demux/9 -> Product5/2  "aq3"
  Iq/1 -> Product5/1, Product/1, Product6/1, Product2/1
  Demux/7 -> Product1/2  "aq1"
  Demux/11 -> Product2/2  "aq5"
  Demux/8 -> Product/2  "aq2"
  Demux/12 -> Product6/2  "aq6"
  Demux/10 -> Product3/2  "aq4"
  Sum2/1 -> Product20/1  "psiq_cross_s1"
  FittingParameters/1 -> Demux/1

== system gm_uz_pmsm_model/Curren t_Controller_With_FluxMaps_OLD/Psi_d_q1/Ldd_approx1 ==
  psiq_cross_s1_integrated : Inport
  Id : Inport  Port=2
  FittingParameters : Inport  Port=3
  Demux : Demux  Outputs=23
  Product{,1..3} (4 alike) : Product  OutDataTypeStr=single
  Product10 : Product  Inputs=3  OutDataTypeStr=single
  Product14 : Product
  Product15 : Product
  Reciprocal : Product  Inputs=/  RndMeth=Zero  SaturateOnIntegerOverflow=on
  Reciprocal1 : Product  Inputs=/  RndMeth=Zero  SaturateOnIntegerOverflow=on
  Sum : Sum  Inputs=|+-  OutDataTypeStr=single
  Sum1 : Sum  Inputs=|+-  OutDataTypeStr=single
  Sum2 : Sum  Inputs=|+-
  Sum7 : Sum  Inputs=|+-
  Tanh1 : Trigonometry  Operator=cosh
  Tanh4 : Trigonometry  Operator=cosh
  Ldd : Outport
  wires:
  Demux/16 -> Product1/2  "ad1*ad2"
  Demux/15 -> Product3/2  "ad4*ad5"
  Reciprocal/1 -> Product1/1
  psiq_cross_s1_integrated/1 -> Product10/2
  Product2/1 -> Tanh1/1
  Product/1 -> Tanh4/1
  Product14/1 -> Reciprocal/1
  Product15/1 -> Reciprocal1/1
  Reciprocal1/1 -> Product3/1
  Tanh1/1 -> Product15/1, Product15/2
  Tanh4/1 -> Product14/2, Product14/1
  Demux/13 -> Product10/3  "F1G1"
  Sum7/1 -> Ldd/1  "psid_cross_s1"
  Product10/1 -> Sum7/2  "psid_cross"
  Sum2/1 -> Product10/1  "psid_cross_s1_abgeleitet"
  Product3/1 -> Sum2/2  "psid_s1"
  Id/1 -> Sum/1, Sum1/1
  Demux/6 -> Sum1/2  "ad6"
  Demux/5 -> Product2/2  "ad5"
  Sum1/1 -> Product2/1
  Product1/1 -> Sum2/1, Sum7/1  "psidself_abgeleitet"
  Demux/2 -> Product/2  "ad2"
  Sum/1 -> Product/1
  Demux/3 -> Sum/2  "ad3"
  FittingParameters/1 -> Demux/1

== system gm_uz_pmsm_model/Curren t_Controller_With_FluxMaps_OLD/Psi_d_q1/Lqq_approx1 ==
  psid_cross_s1_integrated : Inport
  Iq : Inport  Port=2
  FittingParameters : Inport  Port=3
  Demux : Demux  Outputs=23
  Product : Product  OutDataTypeStr=Inherit: Same as first input
  Product1 : Product
  Product14 : Product  OutDataTypeStr=Inherit: Same as first input
  Product15 : Product
  Product2 : Product  OutDataTypeStr=Inherit: Same as first input
  Product20 : Product  Inputs=3
  Product3 : Product
  Reciprocal : Product  Inputs=/  RndMeth=Zero  SaturateOnIntegerOverflow=on
  Reciprocal1 : Product  Inputs=/  RndMeth=Zero  SaturateOnIntegerOverflow=on
  Sum1 : Sum  Inputs=|++
  Sum10 : Sum  Inputs=|+-
  Sum2 : Sum  Inputs=|+-
  Sum4 : Sum  Inputs=|++
  Tanh1 : Trigonometry  Operator=cosh
  Tanh3 : Trigonometry  Operator=cosh
  Lqq : Outport
  wires:
  Demux/17 -> Product3/2  "aq4*aq5"
  Demux/18 -> Product1/2  "aq1*aq2"
  psid_cross_s1_integrated/1 -> Product20/2
  Product14/1 -> Reciprocal/1
  Product/1 -> Tanh3/1
  Product2/1 -> Tanh1/1
  Product15/1 -> Reciprocal1/1
  Product3/1 -> Sum4/1  "psid_s1"
  Sum4/1 -> Sum2/2
  Sum1/1 -> Sum2/1, Sum10/1
  Product1/1 -> Sum1/1  "psidself_abgeleitet"
  Demux/11 -> Product2/2  "aq5"
  Iq/1 -> Product/1, Product2/1
  Demux/8 -> Product/2  "aq2"
  Reciprocal1/1 -> Product3/1
  Reciprocal/1 -> Product1/1
  Sum2/1 -> Product20/1
  Tanh1/1 -> Product15/1, Product15/2
  Tanh3/1 -> Product14/2, Product14/1
  Demux/9 -> Sum1/2  "aq3"
  Demux/14 -> Product20/3
  Sum10/1 -> Lqq/1  "Lqq"
  Product20/1 -> Sum10/2  "psiq_cross"
  Demux/12 -> Sum4/2  "aq6"
  FittingParameters/1 -> Demux/1

== system gm_uz_pmsm_model/Curren t_Controller_With_FluxMaps_OLD/Psi_d_q1/psid_approx ==
  Id : Inport
  Iq : Inport  Port=2
  FittingParameters : Inport  Port=3
  Demux : Demux  Outputs=23
  Log : Math  Operator=log  SignedPower=on
  Log1 : Math  Operator=log  SignedPower=on
  Product{,1..2,4..5,8} (6 alike) : Product  OutDataTypeStr=Inherit: Same as first input
  Product10 : Product  Inputs=3
  Product{3,6..7,12} (4 alike) : Product
  Sum : Sum  Inputs=|+-  OutDataTypeStr=Inherit: Same as first input
  Sum1 : Sum  Inputs=|+-
  Sum2 : Sum  Inputs=|+-  OutDataTypeStr=Inherit: Same as first input
  Sum3 : Sum  Inputs=|++-  OutDataTypeStr=Inherit: Same as first input
  Sum7 : Sum  Inputs=|+-  OutDataTypeStr=Inherit: Same as first input
  Tanh : Trigonometry  Operator=tanh
  Tanh1 : Trigonometry  Operator=tanh
  Tanh2 : Trigonometry  Operator=cosh
  Tanh3 : Trigonometry  Operator=cosh
  Terminator : Terminator
  psid : Outport
  psiq_cross_s1_integrated : Outport  Port=2
  wires:
  Demux/23 -> Product7/2
  Product5/1 -> Tanh3/1
  Product4/1 -> Tanh2/1
  Product2/1 -> Tanh1/1
  Product/1 -> Tanh/1
  Tanh1/1 -> Product3/1
  Tanh/1 -> Product1/1
  Log1/1 -> Product12/1
  Log/1 -> Product6/1
  Demux/13 -> Product10/3  "Reciprodical_F1G1"
  Demux/14 -> Terminator/1
  Sum7/1 -> psid/1  "psi_d_approx"
  Product10/1 -> Sum7/2  "psid_cross"
  Demux/8 -> Product4/2  "aq2"
  Demux/11 -> Product5/2  "aq5"
  Sum3/1 -> psiq_cross_s1_integrated/1, Product10/2  "psiq_cross_s1_integrated"
  Product12/1 -> Sum3/3
  Demux/19 -> Product12/2
  Product6/1 -> Sum3/1
  Demux/20 -> Product6/2
  Product7/1 -> Sum3/2
  Product8/1 -> Product7/1
  Tanh3/1 -> Log1/1
  Tanh2/1 -> Log/1
  Sum2/1 -> Product10/1  "psid_cross_s1"
  Iq/1 -> Product4/1, Product5/1, Product8/1, Product8/2
  Product3/1 -> Sum2/2  "psid_s1"
  Id/1 -> Sum/1, Sum1/1
  Demux/6 -> Sum1/2  "ad6"
  Demux/5 -> Product2/2  "ad5"
  Sum1/1 -> Product2/1
  Demux/4 -> Product3/2  "ad4"
  Product1/1 -> Sum2/1, Sum7/1  "psidself"
  Demux/2 -> Product/2  "ad2"
  Sum/1 -> Product/1
  Demux/3 -> Sum/2  "ad3"
  Demux/1 -> Product1/2  "ad1"
  FittingParameters/1 -> Demux/1

== system gm_uz_pmsm_model/Curren t_Controller_With_FluxMaps_OLD/Psi_d_q1/psiq_approx ==
  Id : Inport
  Iq : Inport  Port=2
  FittingParameters : Inport  Port=3
  Demux : Demux  Outputs=23
  Log1 : Math  Operator=log  SignedPower=on
  Log2 : Math  Operator=log  SignedPower=on
  Product{,2,7,10} (4 alike) : Product  OutDataTypeStr=Inherit: Same as first input
  Product{1,3..6,9} (6 alike) : Product
  Product20 : Product  Inputs=3
  Sum1 : Sum  Inputs=|++
  Sum10 : Sum  Inputs=|+-
  Sum2 : Sum  Inputs=|+-
  Sum3 : Sum  Inputs=-+|
  Sum4 : Sum  Inputs=++|
  Sum5 : Sum  Inputs=|+-
  Sum6 : Sum  Inputs=-+|
  Tanh : Trigonometry  Operator=tanh
  Tanh1 : Trigonometry  Operator=tanh
  Tanh2 : Trigonometry  Operator=cosh
  Tanh4 : Trigonometry  Operator=cosh
  psiq : Outport
  psid_cross_s1_integrated : Outport  Port=2
  wires:
  Product/1 -> Tanh/1
  Product2/1 -> Tanh1/1
  Tanh/1 -> Product1/1
  Tanh1/1 -> Product3/1
  Log2/1 -> Product4/2
  Log1/1 -> Product9/2
  Demux/14 -> Product20/3
  Sum10/1 -> psiq/1  "psiq_approx"
  Product20/1 -> Sum10/2  "psiq_cross"
  Sum5/1 -> Product20/2, psid_cross_s1_integrated/1  "psid_cross_s1_integrated"
  Id/1 -> Sum3/2, Sum6/2
  Demux/6 -> Sum6/1  "ad6"
  Demux/5 -> Product10/1  "ad5"
  Demux/2 -> Product7/1  "ad2"
  Demux/3 -> Sum3/1  "ad3"
  Sum6/1 -> Product10/2  "psid_cross_s1"
  Demux/21 -> Product9/1
  Tanh2/1 -> Log1/1
  Product10/1 -> Tanh2/1  "psid_s1"
  Product9/1 -> Sum5/2
  Product4/1 -> Sum5/1
  Product7/1 -> Tanh4/1  "psid_s1"
  Sum3/1 -> Product7/2  "psid_cross_s1"
  Product6/1 -> Sum1/2
  Product3/1 -> Sum1/1  "psiq_s1"
  Sum1/1 -> Sum2/2
  Sum4/1 -> Sum2/1, Sum10/1  "psiq_self"
  Product5/1 -> Sum4/1
  Product1/1 -> Sum4/2
  Demux/22 -> Product4/1
  Tanh4/1 -> Log2/1
  Demux/9 -> Product5/2  "aq3"
  Iq/1 -> Product5/1, Product/1, Product6/1, Product2/1
  Demux/7 -> Product1/2  "aq1"
  Demux/11 -> Product2/2  "aq5"
  Demux/8 -> Product/2  "aq2"
  Demux/12 -> Product6/2  "aq6"
  Demux/10 -> Product3/2  "aq4"
  Sum2/1 -> Product20/1  "psiq_cross_s1"
  FittingParameters/1 -> Demux/1

== system gm_uz_pmsm_model/Current_Controller1/Entkopplungen/Lineare_Entkopplung ==
  i_d : Inport
  i_q : Inport  Port=2
  omega_m : Inport  Port=3
  Constant1 : Constant  Value=psi_pm  OutDataTypeStr=Inherit: Inherit via back propagation  SampleTime=-1
  Gain : Gain  Gain=L_q
  Gain1 : Gain  Gain=L_d
  Gain2 : Gain  Gain=polepair  OutDataTypeStr=Inherit: Same as input
  Product : Product  OutDataTypeStr=Inherit: Same as first input
  Product1 : Product  OutDataTypeStr=Inherit: Same as first input
  Sum6 : Sum  Inputs=|++
  u_d : Outport
  u_q : Outport  Port=2
  wires:
  Constant1/1 -> Sum6/2  "u_q"
  Gain/1 -> Product/1
  Gain2/1 -> Product/2, Product1/2
  Gain1/1 -> Sum6/1
  Product1/1 -> u_q/1
  i_q/1 -> Gain/1
  i_d/1 -> Gain1/1
  Product/1 -> u_d/1
  Sum6/1 -> Product1/1
  omega_m/1 -> Gain2/1

== system gm_uz_pmsm_model/Current_Controller1/Entkopplungen/decoupling_praediktion ==
  i_d : Inport
  u_d_1 : Inport  Port=2
  i_q : Inport  Port=3
  u_q_1 : Inport  Port=4
  omega_m : Inport  Port=5
  u_d_k : Inport  Port=6
  u_q_k : Inport  Port=7
  psi_q : Inport  Port=8
  psi_d : Inport  Port=9
  Gain : Gain  Gain=R_1
  Gain1 : Gain  Gain=R_1
  Gain2 : Gain  Gain=polepair
  Gain3 : Gain  Gain=ts_regler
  Gain4 : Gain  Gain=ts_regler
  Gain5 : Gain  Gain=ts_regler/2
  Gain6 : Gain  Gain=ts_regler/2
  Product{1..4} (4 alike) : Product
  Sum : Sum  Inputs=|+-
  Sum1 : Sum  Inputs=|+-
  Sum2 : Sum  Inputs=++|
  Sum3 : Sum  Inputs=|-+
  Sum4 : Sum  Inputs=++|
  Sum5 : Sum  Inputs=|++
  Sum6 : Sum  Inputs=++|
  Sum7 : Sum  Inputs=|++
  u_d_entk : Outport
  u_q_entk : Outport  Port=2
  wires:
  Product4/1 -> u_d_entk/1
  Product1/1 -> u_q_entk/1
  i_q/1 -> Gain1/1
  i_d/1 -> Gain/1
  omega_m/1 -> Gain2/1
  Sum7/1 -> Product4/2
  Sum6/1 -> Product1/1
  Gain6/1 -> Sum7/2
  Sum5/1 -> Sum7/1
  Gain5/1 -> Sum6/1
  u_q_1/1 -> Gain6/1
  Sum4/1 -> Sum6/2
  u_d_1/1 -> Gain5/1
  Gain4/1 -> Sum5/1
  Gain3/1 -> Sum4/2
  Sum2/1 -> Gain3/1
  Sum3/1 -> Gain4/1
  Sum1/1 -> Sum3/2
  Sum/1 -> Sum2/1
  Product2/1 -> Sum2/2
  Product3/1 -> Sum3/1
  Gain1/1 -> Sum1/2
  u_q_k/1 -> Sum1/1
  Gain/1 -> Sum/1
  u_d_k/1 -> Sum/2
  Gain2/1 -> Product2/2, Product3/1, Product4/1, Product1/2
  psi_d/1 -> Sum4/1, Product3/2
  psi_q/1 -> Product2/1, Sum5/2

== system gm_uz_pmsm_model/Current_Controller1/Entkopplungen/dynamic_nonlinear_entkopplung1 ==
  i_d : Inport
  i_q : Inport  Port=2
  psi_d : Inport  Port=3
  psi_q : Inport  Port=4
  Ldq_LUT : Inport  Port=5
  Lqd_LUT : Inport  Port=6
  omega_m : Inport  Port=7
  Gain2 : Gain  Gain=polepair
  Product : Product  OutDataTypeStr=Inherit: Same as first input
  Product1 : Product  OutDataTypeStr=Inherit: Same as first input
  Product2 : Product
  Product3 : Product
  Sum1 : Sum  Inputs=++|  OutDataTypeStr=Inherit: Same as first input
  Sum6 : Sum  Inputs=++|
  u_d : Outport
  u_q : Outport  Port=2
  wires:
  Product2/1 -> Sum1/1
  Product3/1 -> Sum6/1
  Lqd_LUT/1 -> Product3/2
  i_q/1 -> Product3/1
  Sum1/1 -> u_d/1
  Product/1 -> Sum1/2
  Product1/1 -> Sum6/2
  Sum6/1 -> u_q/1
  Ldq_LUT/1 -> Product2/2
  i_d/1 -> Product2/1
  omega_m/1 -> Gain2/1
  psi_d/1 -> Product1/1  "psi_d_LUT"
  Gain2/1 -> Product/2, Product1/2
  psi_q/1 -> Product/1  "psi_q_LUT"

== system gm_uz_pmsm_model/Current_Controller1/Entkopplungen/static_nonlinear_entkopplung ==
  psi_d : Inport
  psi_q : Inport  Port=2
  omega_m : Inport  Port=3
  Gain2 : Gain  Gain=polepair
  Product : Product  OutDataTypeStr=Inherit: Same as first input
  Product1 : Product  OutDataTypeStr=Inherit: Same as first input
  u_d : Outport
  u_q : Outport  Port=2
  wires:
  omega_m/1 -> Gain2/1
  psi_d/1 -> Product1/1  "psi_d_LUT"
  Product/1 -> u_d/1
  Product1/1 -> u_q/1
  Gain2/1 -> Product/2, Product1/2
  psi_q/1 -> Product/1  "psi_q_LUT"

== system gm_uz_pmsm_model/Current_Controller1/Psi_d_q1/Ldd_approx1 ==
  psiq_cross_s1_integrated : Inport
  Id : Inport  Port=2
  FittingParameters : Inport  Port=3
  Demux : Demux  Outputs=23
  Product{,1..3} (4 alike) : Product  OutDataTypeStr=single
  Product10 : Product  Inputs=3  OutDataTypeStr=single
  Product14 : Product
  Product15 : Product
  Reciprocal : Product  Inputs=/  RndMeth=Zero  SaturateOnIntegerOverflow=on
  Reciprocal1 : Product  Inputs=/  RndMeth=Zero  SaturateOnIntegerOverflow=on
  Sum : Sum  Inputs=|+-  OutDataTypeStr=single
  Sum1 : Sum  Inputs=|+-  OutDataTypeStr=single
  Sum2 : Sum  Inputs=|+-
  Sum7 : Sum  Inputs=|+-
  Tanh1 : Trigonometry  Operator=cosh
  Tanh4 : Trigonometry  Operator=cosh
  Ldd : Outport
  wires:
  Demux/16 -> Product1/2  "ad1*ad2"
  Demux/15 -> Product3/2  "ad4*ad5"
  Reciprocal/1 -> Product1/1
  psiq_cross_s1_integrated/1 -> Product10/2
  Product2/1 -> Tanh1/1
  Product/1 -> Tanh4/1
  Product14/1 -> Reciprocal/1
  Product15/1 -> Reciprocal1/1
  Reciprocal1/1 -> Product3/1
  Tanh1/1 -> Product15/1, Product15/2
  Tanh4/1 -> Product14/2, Product14/1
  Demux/13 -> Product10/3  "F1G1"
  Sum7/1 -> Ldd/1  "psid_cross_s1"
  Product10/1 -> Sum7/2  "psid_cross"
  Sum2/1 -> Product10/1  "psid_cross_s1_abgeleitet"
  Product3/1 -> Sum2/2  "psid_s1"
  Id/1 -> Sum/1, Sum1/1
  Demux/6 -> Sum1/2  "ad6"
  Demux/5 -> Product2/2  "ad5"
  Sum1/1 -> Product2/1
  Product1/1 -> Sum2/1, Sum7/1  "psidself_abgeleitet"
  Demux/2 -> Product/2  "ad2"
  Sum/1 -> Product/1
  Demux/3 -> Sum/2  "ad3"
  FittingParameters/1 -> Demux/1

== system gm_uz_pmsm_model/Current_Controller1/Psi_d_q1/Lqq_approx1 ==
  psid_cross_s1_integrated : Inport
  Iq : Inport  Port=2
  FittingParameters : Inport  Port=3
  Demux : Demux  Outputs=23
  Product : Product  OutDataTypeStr=Inherit: Same as first input
  Product1 : Product
  Product14 : Product  OutDataTypeStr=Inherit: Same as first input
  Product15 : Product
  Product2 : Product  OutDataTypeStr=Inherit: Same as first input
  Product20 : Product  Inputs=3
  Product3 : Product
  Reciprocal : Product  Inputs=/  RndMeth=Zero  SaturateOnIntegerOverflow=on
  Reciprocal1 : Product  Inputs=/  RndMeth=Zero  SaturateOnIntegerOverflow=on
  Sum1 : Sum  Inputs=|++
  Sum10 : Sum  Inputs=|+-
  Sum2 : Sum  Inputs=|+-
  Sum4 : Sum  Inputs=|++
  Tanh1 : Trigonometry  Operator=cosh
  Tanh3 : Trigonometry  Operator=cosh
  Lqq : Outport
  wires:
  Demux/17 -> Product3/2  "aq4*aq5"
  Demux/18 -> Product1/2  "aq1*aq2"
  psid_cross_s1_integrated/1 -> Product20/2
  Product14/1 -> Reciprocal/1
  Product/1 -> Tanh3/1
  Product2/1 -> Tanh1/1
  Product15/1 -> Reciprocal1/1
  Product3/1 -> Sum4/1  "psid_s1"
  Sum4/1 -> Sum2/2
  Sum1/1 -> Sum2/1, Sum10/1
  Product1/1 -> Sum1/1  "psidself_abgeleitet"
  Demux/11 -> Product2/2  "aq5"
  Iq/1 -> Product/1, Product2/1
  Demux/8 -> Product/2  "aq2"
  Reciprocal1/1 -> Product3/1
  Reciprocal/1 -> Product1/1
  Sum2/1 -> Product20/1
  Tanh1/1 -> Product15/1, Product15/2
  Tanh3/1 -> Product14/2, Product14/1
  Demux/9 -> Sum1/2  "aq3"
  Demux/14 -> Product20/3
  Sum10/1 -> Lqq/1  "Lqq"
  Product20/1 -> Sum10/2  "psiq_cross"
  Demux/12 -> Sum4/2  "aq6"
  FittingParameters/1 -> Demux/1

== system gm_uz_pmsm_model/Current_Controller1/Psi_d_q1/psid_approx ==
  Id : Inport
  Iq : Inport  Port=2
  FittingParameters : Inport  Port=3
  Demux : Demux  Outputs=23
  Log : Math  Operator=log  SignedPower=on
  Log1 : Math  Operator=log  SignedPower=on
  Product{,1..2,4..5,8} (6 alike) : Product  OutDataTypeStr=Inherit: Same as first input
  Product10 : Product  Inputs=3
  Product{3,6..7,12} (4 alike) : Product
  Sum : Sum  Inputs=|+-  OutDataTypeStr=Inherit: Same as first input
  Sum1 : Sum  Inputs=|+-
  Sum2 : Sum  Inputs=|+-  OutDataTypeStr=Inherit: Same as first input
  Sum3 : Sum  Inputs=|++-  OutDataTypeStr=Inherit: Same as first input
  Sum7 : Sum  Inputs=|+-  OutDataTypeStr=Inherit: Same as first input
  Tanh : Trigonometry  Operator=tanh
  Tanh1 : Trigonometry  Operator=tanh
  Tanh2 : Trigonometry  Operator=cosh
  Tanh3 : Trigonometry  Operator=cosh
  Terminator : Terminator
  psid : Outport
  psiq_cross_s1_integrated : Outport  Port=2
  wires:
  Demux/23 -> Product7/2
  Product5/1 -> Tanh3/1
  Product4/1 -> Tanh2/1
  Product2/1 -> Tanh1/1
  Product/1 -> Tanh/1
  Tanh1/1 -> Product3/1
  Tanh/1 -> Product1/1
  Log1/1 -> Product12/1
  Log/1 -> Product6/1
  Demux/13 -> Product10/3  "Reciprodical_F1G1"
  Demux/14 -> Terminator/1
  Sum7/1 -> psid/1  "psi_d_approx"
  Product10/1 -> Sum7/2  "psid_cross"
  Demux/8 -> Product4/2  "aq2"
  Demux/11 -> Product5/2  "aq5"
  Sum3/1 -> psiq_cross_s1_integrated/1, Product10/2  "psiq_cross_s1_integrated"
  Product12/1 -> Sum3/3
  Demux/19 -> Product12/2
  Product6/1 -> Sum3/1
  Demux/20 -> Product6/2
  Product7/1 -> Sum3/2
  Product8/1 -> Product7/1
  Tanh3/1 -> Log1/1
  Tanh2/1 -> Log/1
  Sum2/1 -> Product10/1  "psid_cross_s1"
  Iq/1 -> Product4/1, Product5/1, Product8/1, Product8/2
  Product3/1 -> Sum2/2  "psid_s1"
  Id/1 -> Sum/1, Sum1/1
  Demux/6 -> Sum1/2  "ad6"
  Demux/5 -> Product2/2  "ad5"
  Sum1/1 -> Product2/1
  Demux/4 -> Product3/2  "ad4"
  Product1/1 -> Sum2/1, Sum7/1  "psidself"
  Demux/2 -> Product/2  "ad2"
  Sum/1 -> Product/1
  Demux/3 -> Sum/2  "ad3"
  Demux/1 -> Product1/2  "ad1"
  FittingParameters/1 -> Demux/1

== system gm_uz_pmsm_model/Current_Controller1/Psi_d_q1/psiq_approx ==
  Id : Inport
  Iq : Inport  Port=2
  FittingParameters : Inport  Port=3
  Demux : Demux  Outputs=23
  Log1 : Math  Operator=log  SignedPower=on
  Log2 : Math  Operator=log  SignedPower=on
  Product{,2,7,10} (4 alike) : Product  OutDataTypeStr=Inherit: Same as first input
  Product{1,3..6,9} (6 alike) : Product
  Product20 : Product  Inputs=3
  Sum1 : Sum  Inputs=|++
  Sum10 : Sum  Inputs=|+-
  Sum2 : Sum  Inputs=|+-
  Sum3 : Sum  Inputs=-+|
  Sum4 : Sum  Inputs=++|
  Sum5 : Sum  Inputs=|+-
  Sum6 : Sum  Inputs=-+|
  Tanh : Trigonometry  Operator=tanh
  Tanh1 : Trigonometry  Operator=tanh
  Tanh2 : Trigonometry  Operator=cosh
  Tanh4 : Trigonometry  Operator=cosh
  psiq : Outport
  psid_cross_s1_integrated : Outport  Port=2
  wires:
  Product/1 -> Tanh/1
  Product2/1 -> Tanh1/1
  Tanh/1 -> Product1/1
  Tanh1/1 -> Product3/1
  Log2/1 -> Product4/2
  Log1/1 -> Product9/2
  Demux/14 -> Product20/3
  Sum10/1 -> psiq/1  "psiq_approx"
  Product20/1 -> Sum10/2  "psiq_cross"
  Sum5/1 -> Product20/2, psid_cross_s1_integrated/1  "psid_cross_s1_integrated"
  Id/1 -> Sum3/2, Sum6/2
  Demux/6 -> Sum6/1  "ad6"
  Demux/5 -> Product10/1  "ad5"
  Demux/2 -> Product7/1  "ad2"
  Demux/3 -> Sum3/1  "ad3"
  Sum6/1 -> Product10/2  "psid_cross_s1"
  Demux/21 -> Product9/1
  Tanh2/1 -> Log1/1
  Product10/1 -> Tanh2/1  "psid_s1"
  Product9/1 -> Sum5/2
  Product4/1 -> Sum5/1
  Product7/1 -> Tanh4/1  "psid_s1"
  Sum3/1 -> Product7/2  "psid_cross_s1"
  Product6/1 -> Sum1/2
  Product3/1 -> Sum1/1  "psiq_s1"
  Sum1/1 -> Sum2/2
  Sum4/1 -> Sum2/1, Sum10/1  "psiq_self"
  Product5/1 -> Sum4/1
  Product1/1 -> Sum4/2
  Demux/22 -> Product4/1
  Tanh4/1 -> Log2/1
  Demux/9 -> Product5/2  "aq3"
  Iq/1 -> Product5/1, Product/1, Product6/1, Product2/1
  Demux/7 -> Product1/2  "aq1"
  Demux/11 -> Product2/2  "aq5"
  Demux/8 -> Product/2  "aq2"
  Demux/12 -> Product6/2  "aq6"
  Demux/10 -> Product3/2  "aq4"
  Sum2/1 -> Product20/1  "psiq_cross_s1"
  FittingParameters/1 -> Demux/1

== system gm_uz_pmsm_model/Current_Controller_With_FluxMaps_OLD1/Entkopplungen/Lineare_Entkopplung ==
  i_d : Inport
  i_q : Inport  Port=2
  omega_m : Inport  Port=3
  Constant1 : Constant  Value=psi_pm  SampleTime=-1
  Gain : Gain  Gain=L_q
  Gain1 : Gain  Gain=L_d
  Gain2 : Gain  Gain=polepair
  Product : Product
  Product1 : Product
  Sum6 : Sum  Inputs=|++
  u_d : Outport
  u_q : Outport  Port=2
  wires:
  Gain/1 -> Product/1
  Gain2/1 -> Product/2, Product1/2
  Gain1/1 -> Sum6/1
  Product1/1 -> u_q/1
  i_q/1 -> Gain/1
  Constant1/1 -> Sum6/2
  i_d/1 -> Gain1/1
  Product/1 -> u_d/1
  Sum6/1 -> Product1/1
  omega_m/1 -> Gain2/1

== system gm_uz_pmsm_model/Current_Controller_With_FluxMaps_OLD1/Entkopplungen/decoupling_praediktion ==
  i_d : Inport
  u_d_1 : Inport  Port=2
  i_q : Inport  Port=3
  u_q_1 : Inport  Port=4
  omega_m : Inport  Port=5
  u_d_k : Inport  Port=6
  u_q_k : Inport  Port=7
  psi_q : Inport  Port=8
  psi_d : Inport  Port=9
  Gain : Gain  Gain=R_1
  Gain1 : Gain  Gain=R_1
  Gain2 : Gain  Gain=polepair
  Gain3 : Gain  Gain=ts_regler
  Gain4 : Gain  Gain=ts_regler
  Gain5 : Gain  Gain=ts_regler/2
  Gain6 : Gain  Gain=ts_regler/2
  Product{1..4} (4 alike) : Product
  Sum : Sum  Inputs=|+-
  Sum1 : Sum  Inputs=|+-
  Sum2 : Sum  Inputs=++|
  Sum3 : Sum  Inputs=|-+
  Sum4 : Sum  Inputs=++|
  Sum5 : Sum  Inputs=|++
  Sum6 : Sum  Inputs=++|
  Sum7 : Sum  Inputs=|++
  u_d_entk : Outport
  u_q_entk : Outport  Port=2
  wires:
  Product4/1 -> u_d_entk/1
  Product1/1 -> u_q_entk/1
  i_q/1 -> Gain1/1
  i_d/1 -> Gain/1
  omega_m/1 -> Gain2/1
  Sum7/1 -> Product4/2
  Sum6/1 -> Product1/1
  Gain6/1 -> Sum7/2
  Sum5/1 -> Sum7/1
  Gain5/1 -> Sum6/1
  u_q_1/1 -> Gain6/1
  Sum4/1 -> Sum6/2
  u_d_1/1 -> Gain5/1
  Gain4/1 -> Sum5/1
  Gain3/1 -> Sum4/2
  Sum2/1 -> Gain3/1
  Sum3/1 -> Gain4/1
  Sum1/1 -> Sum3/2
  Sum/1 -> Sum2/1
  Product2/1 -> Sum2/2
  Product3/1 -> Sum3/1
  Gain1/1 -> Sum1/2
  u_q_k/1 -> Sum1/1
  Gain/1 -> Sum/1
  u_d_k/1 -> Sum/2
  Gain2/1 -> Product2/2, Product3/1, Product4/1, Product1/2
  psi_d/1 -> Sum4/1, Product3/2
  psi_q/1 -> Product2/1, Sum5/2

== system gm_uz_pmsm_model/Current_Controller_With_FluxMaps_OLD1/Entkopplungen/dynamic_nonlinear_entkopplung1 ==
  i_d : Inport
  i_q : Inport  Port=2
  psi_d : Inport  Port=3
  psi_q : Inport  Port=4
  Ldq_LUT : Inport  Port=5
  Lqd_LUT : Inport  Port=6
  omega_m : Inport  Port=7
  Gain2 : Gain  Gain=polepair
  Product{,1..3} (4 alike) : Product
  Sum1 : Sum  Inputs=++|
  Sum6 : Sum  Inputs=++|
  u_d : Outport
  u_q : Outport  Port=2
  wires:
  Product2/1 -> Sum1/1
  Product3/1 -> Sum6/1
  Lqd_LUT/1 -> Product3/2
  i_q/1 -> Product3/1
  Sum1/1 -> u_d/1
  Product/1 -> Sum1/2
  Product1/1 -> Sum6/2
  Sum6/1 -> u_q/1
  Ldq_LUT/1 -> Product2/2
  i_d/1 -> Product2/1
  omega_m/1 -> Gain2/1
  psi_d/1 -> Product1/1  "psi_d_LUT"
  Gain2/1 -> Product/2, Product1/2
  psi_q/1 -> Product/1  "psi_q_LUT"

== system gm_uz_pmsm_model/Current_Controller_With_FluxMaps_OLD1/Entkopplungen/static_nonlinear_entkopplung ==
  psi_d : Inport
  psi_q : Inport  Port=2
  omega_m : Inport  Port=3
  Gain2 : Gain  Gain=polepair
  Product : Product
  Product1 : Product
  Scope : Scope  NumInputPorts=2
  u_d : Outport
  u_q : Outport  Port=2
  wires:
  omega_m/1 -> Gain2/1
  psi_d/1 -> Product1/1  "psi_d_LUT"
  Product/1 -> u_d/1, Scope/2
  Product1/1 -> u_q/1, Scope/1
  Gain2/1 -> Product/2, Product1/2
  psi_q/1 -> Product/1  "psi_q_LUT"
